simulink library "FAM_quasi_static_outflow_v2"  (R2024a)
settings: Solver=VariableStepAuto  StartTime=0.0  StopTime=10.0  RelTol=1e-3
undefined symbols (not defined in the file): G, kT, kV, power_avg_start_time, R_load, Rm, turbine_D
libraries: simulink x1
settings Model: Creator=Carson  LastModifiedBy=cmmcguir
settings RTWCC: GPUComputeCapability=3.5

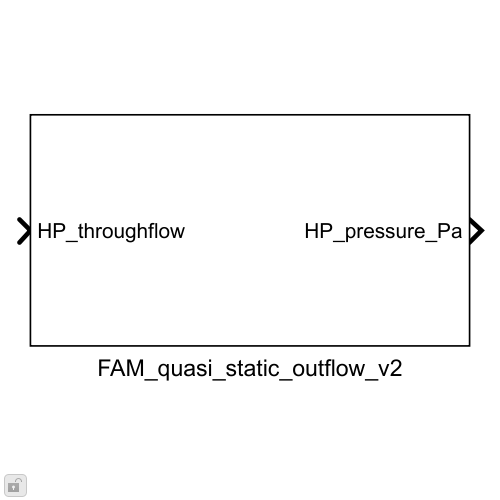
[thumbnail: Simulink's stored preview of the top-level diagram]
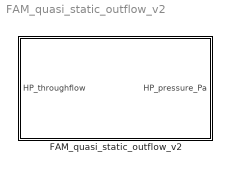
== system FAM_quasi_static_outflow_v2 ==
  FAM_quasi_static_outflow_v2 : Subsystem

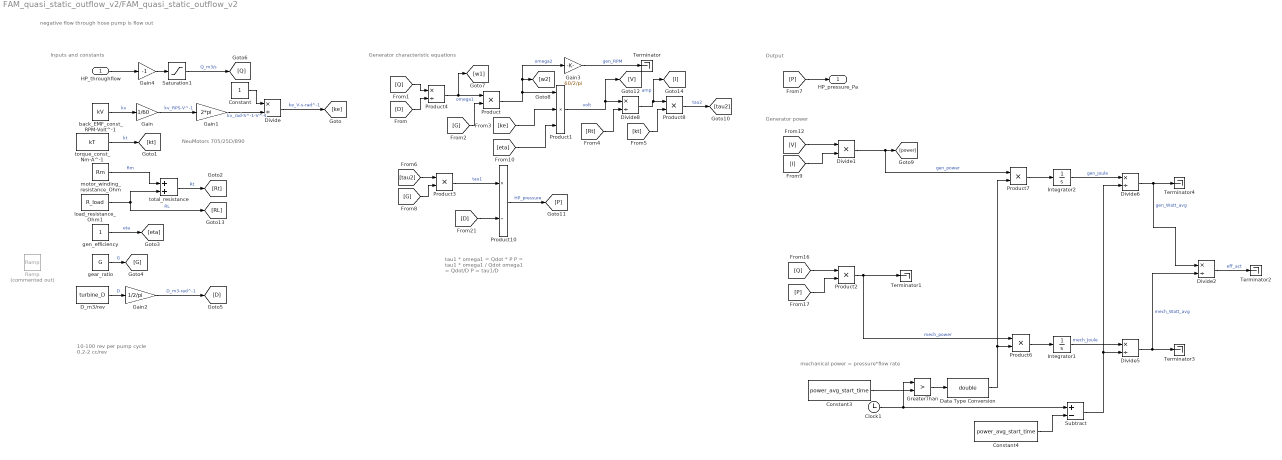
== system FAM_quasi_static_outflow_v2/FAM_quasi_static_outflow_v2 ==
  note: tau1 * omega1 = Qdot * P
      | P = tau1 * omega1 / Qdot
      | 	omega1 = Qdot/D
      | P = tau1/D
  note: NeuMotors 705/25D/890
  note: mechanical power = pressure*flow rate
  note: 10-100 rev per pump cycle
      | 0.2-2 cc/rev
  note: Generator power
  note: Output
  note: Generator characteristic equations
  note: Inputs and constants
  note: negative flow through hose pump is flow out
  HP_throughflow : Inport
  Clock1 : Clock
  Constant : Constant
  Constant3 : Constant  Value=power_avg_start_time
  Constant4 : Constant  Value=power_avg_start_time
  D_m3/rev : Constant  Value=turbine_D
  Data Type Conversion : DataTypeConversion  OutDataTypeStr=double  SaturateOnIntegerOverflow=off  RndMeth=Floor
  Divide{,2,5..6,8} (5 alike) : Product  Inputs=*/
  Divide1 : Product  Inputs=**
  Gain : Gain  Gain=1/60
  Gain1 : Gain  Gain=2*pi
  Gain2 : Gain  Gain=1/2/pi
  Gain3 : Gain  Gain=60/2/pi
  Gain4 : Gain  Gain=-1
  GreaterThan : RelationalOperator  Operator=>  OutDataTypeStr=boolean  RndMeth=Simplest  InputSameDT=off
  Integrator1 : Integrator  ZeroCross=off
  Integrator2 : Integrator
  Product{,2..3,6..8} (6 alike) : Product
  Product1 : Product  Inputs=3
  Product10 : Product  Inputs=*/
  Product4 : Product  Inputs=*/
  Ramp : simulink/Sources/Ramp  Commented=on  slope=0.1  start=60  InitialOutput=1
  Saturation1 : Saturate  UpperLimit=inf  LowerLimit=0
  Subtract : Sum  Inputs=+-
  Terminator{,1..4} (5 alike) : Terminator
  back_EMF_const_RPM-Volt^-1 : Constant  Value=kV
  gear_ratio : Constant  Value=G
  gen_efficiency : Constant
  load_resistance_Ohm1 : Constant  Value=R_load
  motor_winding_resistance_Ohm : Constant  Value=Rm
  torque_const_Nm-A^-1 : Constant  Value=kT
  total_resistance : Sum
  HP_pressure_Pa : Outport
  wires:
  HP_throughflow/1 -> Gain4/1
  torque_const_Nm-A^-1/1 -> [kt]  "kt"
  gen_efficiency/1 -> [eta]  "eta"
  motor_winding_resistance_Ohm/1 -> total_resistance/1  "Rm"
  load_resistance_Ohm1/1 -> total_resistance/2, [RL]  "RL"
  total_resistance/1 -> [Rt]  "Rt"
  Gain/1 -> Gain1/1  "kv_RPS-V^-1"
  Gain1/1 -> Divide/2  "kv_rad-S^-1-V^-1"
  Constant/1 -> Divide/1
  Divide/1 -> [ke]  "ke_V-s-rad^-1"
  D_m3/rev/1 -> Gain2/1  "D"
  Gain2/1 -> [D]  "D_m3-rad^-1"
  [P] -> HP_pressure_Pa/1
  [V] -> Divide1/1
  Divide1/1 -> Product7/1, [power]  "gen_power"
  [Q] -> Product2/1
  [P] -> Product2/2
  Product2/1 -> Product6/1, Terminator1/1  "mech_power"
  back_EMF_const_RPM-Volt^-1/1 -> Gain/1  "kv"
  Divide5/1 -> Divide2/2, Terminator3/1  "mech_Watt_avg"
  Integrator1/1 -> Divide5/1  "mech_Joule"
  gear_ratio/1 -> [G]  "G"
  Divide6/1 -> Divide2/1, Terminator4/1  "gen_Watt_avg"
  Integrator2/1 -> Divide6/1  "gen_Joule"
  Clock1/1 -> Subtract/1, GreaterThan/1
  GreaterThan/1 -> Data Type Conversion/1
  Constant3/1 -> GreaterThan/2
  Data Type Conversion/1 -> Product6/2, Product7/2
  Product6/1 -> Integrator1/1
  Constant4/1 -> Subtract/2
  Subtract/1 -> Divide6/2, Divide5/2
  Product7/1 -> Integrator2/1
  Gain4/1 -> Saturation1/1
  [Q] -> Product4/1
  [D] -> Product4/2
  Product4/1 -> [w1], Product/1  "omega1"
  [G] -> Product/2
  Product/1 -> Gain3/1, [w2], Product1/1  "omega2"
  [ke] -> Product1/2
  Product1/1 -> [V], Divide8/1  "volt"
  [Rt] -> Divide8/2
  Divide8/1 -> [I], Product8/1  "amp"
  [kt] -> Product8/2
  Product8/1 -> [tau2]  "tau2"
  [tau2] -> Product3/1
  Product3/1 -> Product10/1  "tau1"
  [eta] -> Product1/3
  [D] -> Product10/2
  Product10/1 -> [P]  "HP_pressure"
  Saturation1/1 -> [Q]  "Q_m3/s"
  Divide2/1 -> Terminator2/1  "eff_act"
  [G] -> Product3/2
  Gain3/1 -> Terminator/1  "gen_RPM"
  [I] -> Divide1/2
